simulink model "test_connection"  (R2020a)
settings: Solver=FixedStepAuto  StartTime=0.0  StopTime=inf  FixedStep=1e-3  RelTol=1e-3
libraries: powerlib_meascontrol x2, vrlib x1
settings Model: Creator=lucia  LastModifiedBy=lucia
settings DebuggingCC: UnderSpecifiedDimensionMsg=warning

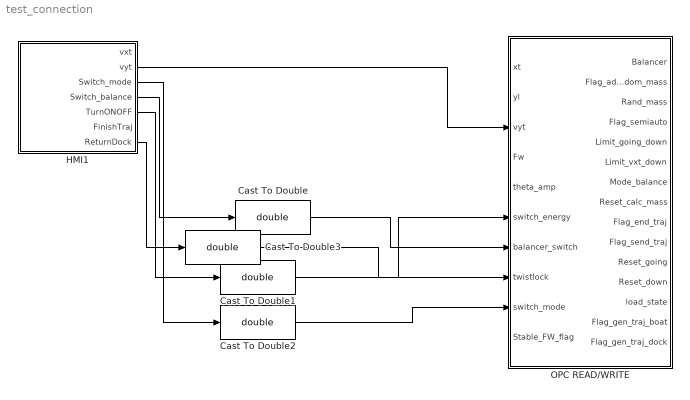
== system test_connection ==
  Cast To Double{,1..3} (4 alike) : DataTypeConversion  OutDataTypeStr=double
  HMI1 : Subsystem
  OPC READ/WRITE : Subsystem  TreatAsAtomicUnit=on  SystemSampleTime=0.1
  wires:
  HMI1/2(vyt) -> OPC READ/WRITE/3(vyt)
  HMI1/3(Switch_mode) -> Cast To Double2/1
  HMI1/4(Switch_balance) -> Cast To Double/1
  HMI1/5(TurnONOFF) -> Cast To Double1/1
  Cast To Double/1 -> OPC READ/WRITE/7(balancer_switch)
  Cast To Double1/1 -> OPC READ/WRITE/6(switch_energy)
  Cast To Double2/1 -> OPC READ/WRITE/9(switch_mode)
  HMI1/7(ReturnDock) -> Cast To Double3/1
  Cast To Double3/1 -> OPC READ/WRITE/8(twistlock)

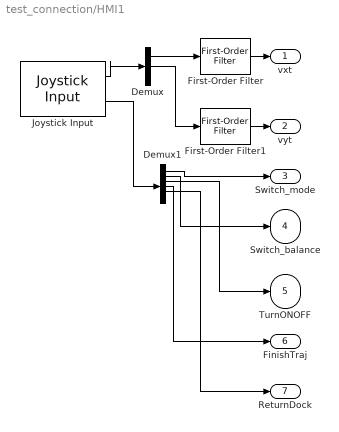
== system test_connection/HMI1 ==
  Demux : Demux  Outputs=3
  Demux1 : Demux  Outputs=6
  First-Order Filter : powerlib_meascontrol/Filters/First-Order Filter  FilterType=Lowpass  Tc=10e-3  Ts=0  Initialize=off  Vac_Init=[0, 0, 60]  Vdc_Init=0  PlotResponse=off  FreqRange="[0,  200,  1]"
  First-Order Filter1 : powerlib_meascontrol/Filters/First-Order Filter  FilterType=Lowpass  Tc=10e-3  Ts=0  Initialize=off  Vac_Init=[0, 0, 60]  Vdc_Init=0  PlotResponse=off  FreqRange="[0,  200,  1]"
  Joystick Input : vrlib/Joystick Input  joyid=1  adjustports=on  forcefeed=off
  vxt : Outport
  vyt : Outport  Port=2
  Switch_mode : Outport  Port=3
  Switch_balance : Outport  Port=4
  TurnONOFF : Outport  Port=5
  FinishTraj : Outport  Port=6
  ReturnDock : Outport  Port=7
  wires:
  Demux1/5 -> ReturnDock/1
  Demux1/4 -> FinishTraj/1
  Demux1/3 -> TurnONOFF/1
  Demux/2 -> First-Order Filter1/1
  Demux/1 -> First-Order Filter/1
  Joystick Input/1 -> Demux/1
  Demux1/1 -> Switch_mode/1
  Joystick Input/2 -> Demux1/1
  Demux1/2 -> Switch_balance/1
  First-Order Filter/1 -> vxt/1
  First-Order Filter1/1 -> vyt/1

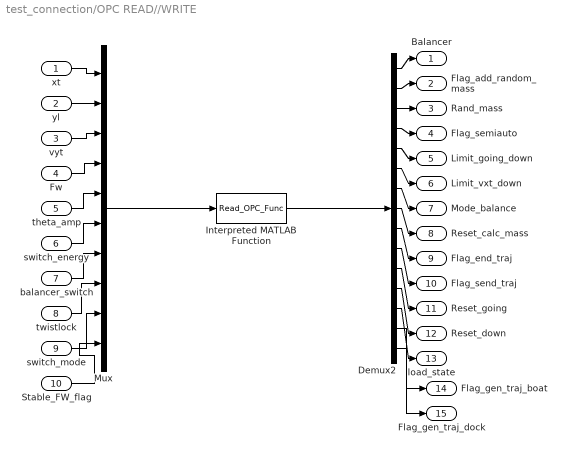
== system test_connection/OPC READ//WRITE ==
  xt : Inport
  yl : Inport  Port=2
  vyt : Inport  Port=3
  Fw : Inport  Port=4
  theta_amp : Inport  Port=5
  switch_energy : Inport  Port=6
  balancer_switch : Inport  Port=7
  twistlock : Inport  Port=8
  switch_mode : Inport  Port=9
  Stable_FW_flag : Inport  Port=10
  Demux2 : Demux  Outputs=15
  Interpreted MATLAB Function : MATLABFcn  MATLABFcn=Read_OPC_Func
  Mux : Mux  Inputs=10
  Balancer : Outport
  Flag_add_random_mass : Outport  Port=2
  Rand_mass : Outport  Port=3
  Flag_semiauto : Outport  Port=4
  Limit_going_down : Outport  Port=5
  Limit_vxt_down : Outport  Port=6
  Mode_balance : Outport  Port=7
  Reset_calc_mass : Outport  Port=8
  Flag_end_traj : Outport  Port=9
  Flag_send_traj : Outport  Port=10
  Reset_going : Outport  Port=11
  Reset_down : Outport  Port=12
  load_state : Outport  Port=13
  Flag_gen_traj_boat : Outport  Port=14
  Flag_gen_traj_dock : Outport  Port=15
  wires:
  Interpreted MATLAB Function/1 -> Demux2/1
  Stable_FW_flag/1 -> Mux/10
  switch_mode/1 -> Mux/9
  twistlock/1 -> Mux/8
  balancer_switch/1 -> Mux/7
  switch_energy/1 -> Mux/6
  Demux2/13 -> load_state/1
  Demux2/2 -> Flag_add_random_mass/1
  Demux2/12 -> Reset_down/1
  Demux2/11 -> Reset_going/1
  Demux2/9 -> Flag_end_traj/1
  Demux2/7 -> Mode_balance/1
  Demux2/3 -> Rand_mass/1
  Demux2/5 -> Limit_going_down/1
  Demux2/6 -> Limit_vxt_down/1
  Demux2/1 -> Balancer/1
  yl/1 -> Mux/2
  Mux/1 -> Interpreted MATLAB Function/1
  xt/1 -> Mux/1
  Demux2/8 -> Reset_calc_mass/1
  vyt/1 -> Mux/3
  Demux2/10 -> Flag_send_traj/1
  theta_amp/1 -> Mux/5
  Fw/1 -> Mux/4
  Demux2/4 -> Flag_semiauto/1
  Demux2/14 -> Flag_gen_traj_boat/1
  Demux2/15 -> Flag_gen_traj_dock/1
